simulink model "Motor_Control_Simulink"  (R2026a)
settings: Solver=VariableStepAuto  StopTime=inf
libraries: instrumentseriallib x2
settings Model: Creator=PC  LastModifiedBy=PC

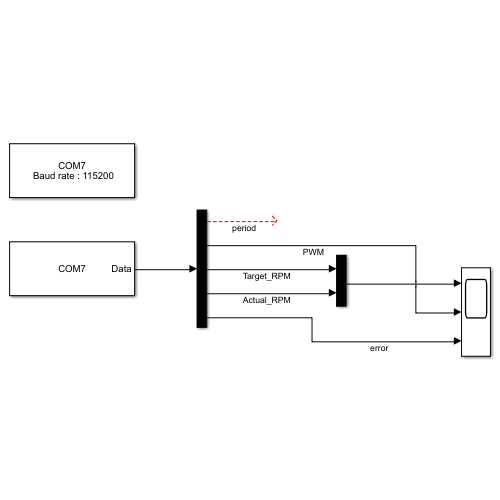
[thumbnail: Simulink's stored preview of the top-level diagram]
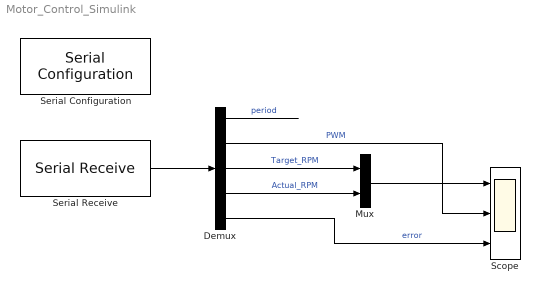
== system Motor_Control_Simulink ==
  Demux : Demux  Outputs=5
  Mux : Mux  Inputs=2
  Scope : Scope  NumInputPorts=3
      settings: TimeSpan=10  Title=RPM  ActiveDisplayYMinimum=-8.5562535990824244  ActiveDisplayYMaximum=338.73124640091805
  Serial Configuration : instrumentseriallib/Serial Configuration  Priority=-200000  PortSel=COM7  Port=COM7  ComPort=COM7  BaudRate=115200  DataBits=8  Parity=none  StopBits=1  ByteOrder=little-endian  FlowControl=none  Timeout=10  SimulateUsing=Interpreted execution  BlockInModel=on  aMode=1
  Serial Receive : instrumentseriallib/Serial Receive  Priority=1  PortSel=COM7  Port=COM7  ComPort=COM7  DataType=single  SaveDataType=uint8  ToggleHeader=on  Header=[170 187]  ToggleDataSize=on  DataSize=5  ToggleTerminator=on  Terminator=<none>  CustomTerminator=[]  InputFormat=Column major  EnableBlockingMode=on  ActionDataUnavailable=Output last received value  ActionWhenDataUnavailable=Output last received value  CustomValue=0  SampleTime=0.05  SimulateUsing=Interpreted execution  BlockInModel=on  aMode=1  LibraryInUse=instrumentlib
  wires:
  Serial Receive/1 -> Demux/1
  Demux/2 -> Scope/2  "PWM"
  Demux/3 -> Mux/1  "Target_RPM"
  Demux/4 -> Mux/2  "Actual_RPM"
  Mux/1 -> Scope/1
  Demux/1 -> ?  "period"
  Demux/5 -> Scope/3  "error"
